simulink model "lista2_prey_pred"  (R2022b)
settings: Solver=FixedStepAuto  StartTime=0.0  StopTime=20.0  FixedStep=0.001  RelTol=1e-3
settings Model: Creator=mateu  LastModifiedBy=mateu

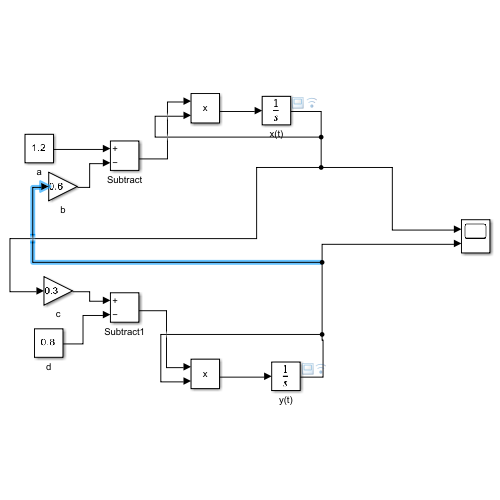
[thumbnail: Simulink's stored preview of the top-level diagram]
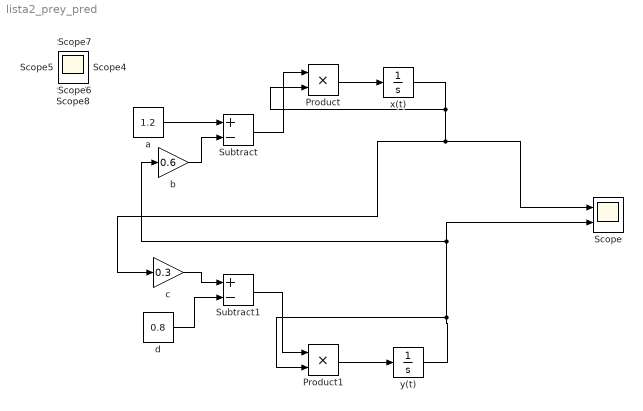
== system lista2_prey_pred ==
  Product : Product
  Product1 : Product
  Scope : Scope  NumInputPorts=2
  Subtract : Sum  Inputs=+-
  Subtract1 : Sum  Inputs=+-
  a : Constant  Value=1.2
  b : Gain  Gain=0.6
  c : Gain  Gain=0.3
  d : Constant  Value=0.8
  x(t) : Integrator  InitialCondition=2
  y(t) : Integrator  InitialCondition=1
  Scope{1..8} (8 alike) : Scope
  wires:
  x(t)/1 -> Scope/1, c/1, Product/2
  y(t)/1 -> Scope/2, b/1, Product1/2
  c/1 -> Subtract1/1
  d/1 -> Subtract1/2
  Subtract1/1 -> Product1/1
  a/1 -> Subtract/1
  b/1 -> Subtract/2
  Subtract/1 -> Product/1
  Product/1 -> x(t)/1
  Product1/1 -> y(t)/1
